simulink model "CPU 4 bit"  (R2022b)
settings: Solver=FixedStepDiscrete  StartTime=0.0  StopTime=10.0  RelTol=1e-3
libraries: hdlsllib x91
settings Model: DataTypeOverride=Off  Creator=canti  LastModifiedBy=canti
settings SolverCC: AlgebraicLoopSolver=TrustRegion
settings DataIOCC: LimitDataPoints=on  SaveOutput=off  SaveTime=off
settings OptimizationCC: BlockReduction=off  ConditionallyExecuteInputs=off  DefaultParameterBehavior=Inlined  LifeSpan=inf
settings DebuggingCC: AlgebraicLoopMsg=error  SingleTaskRateTransMsg=error  UnconnectedInputMsg=warning  UnconnectedOutputMsg=warning  UnconnectedLineMsg=warning  AllowSymbolicDim=off  StrictBusMsg=ErrorOnBusTreatedAsVector  SFUnexpectedBacktrackingDiag=warning  SFNoUnconditionalDefaultTransitionDiag=warning  SFExecutionAtInitializationDiag=none  SFMachineParentedDataDiag=warning  ArithmeticOperatorsInVariantConditions=warning
settings HardwareCC: ProdBitPerPointer=32  ProdBitPerSizeT=32  ProdBitPerPtrDiffT=32  ProdLargestAtomicFloat=None  ProdIntDivRoundTo=Undefined  ProdEndianess=Unspecified  ProdWordSize=32  ProdHWDeviceType=ASIC/FPGA->ASIC/FPGA  ProdEqTarget=off
settings ModelReferenceCC: EnableRefExpFcnMdlSchedulingChecks=on
settings SFSimCC: SimUseLocalCustomCode=off  CustomCodeUndefinedFunction=UseInterfaceOnly
settings RTWCC: RTWUseLocalCustomCode=off
settings CodeAppCC: StateflowObjectComments=on
settings GRTTargetCC: TargetLangStandard=C89/C90 (ANSI)
settings ConfigComp: CovScope=ReferencedModels  CovMetricSettings=dw  CovSaveCumulativeToWorkspaceVar=on  CovSaveSingleToWorkspaceVar=on  CovExternalEMLEnable=off  CovSFcnEnable=off

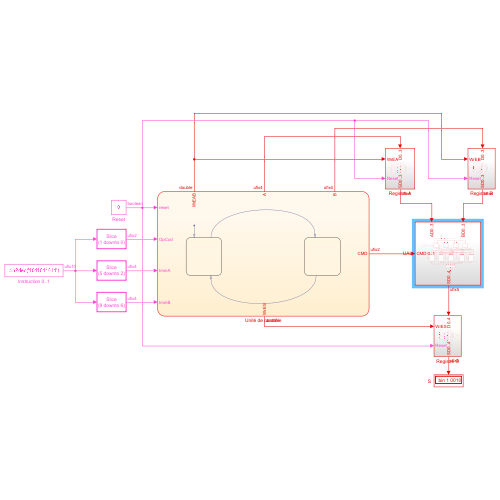
[thumbnail: Simulink's stored preview of the top-level diagram]
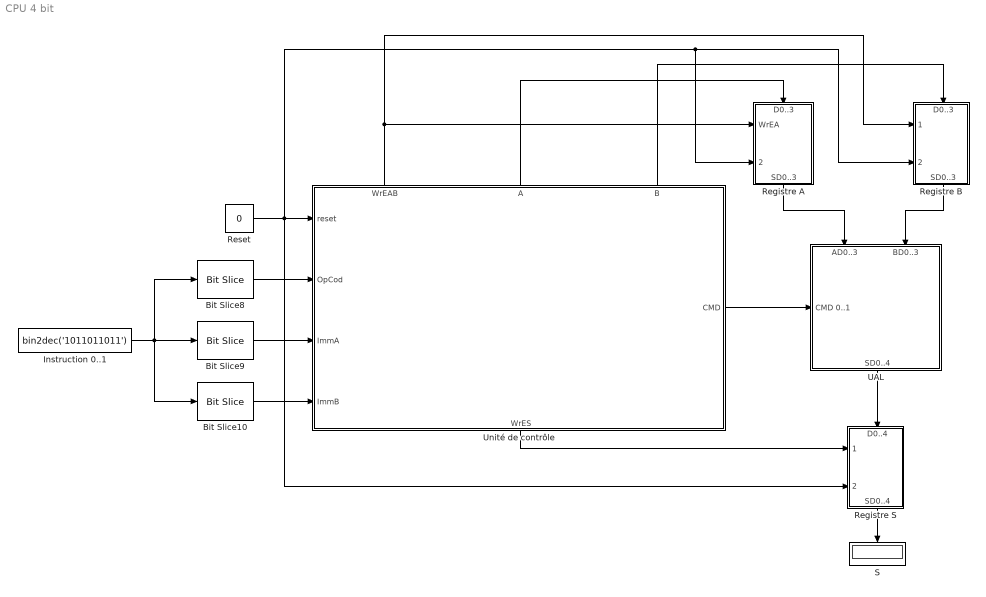
== system CPU 4 bit ==
  Bit Slice10 : hdlsllib/Logic and Bit Operations/Bit Slice  lidx=9  ridx=6
  Bit Slice8 : hdlsllib/Logic and Bit Operations/Bit Slice  lidx=1  ridx=0
  Bit Slice9 : hdlsllib/Logic and Bit Operations/Bit Slice  lidx=5  ridx=2
  Instruction 0..1 : Constant  Value=bin2dec('1011011011')  VectorParams1D=off  OutDataTypeStr=fixdt(0,10,0)
  Registre A : Subsystem
      settings: PortSchema="{\"entries\":[{\"content\":{\"sides\":[{\"content\":{\"connectorIds\":[\"In1\",\"In2\"]},\"type\":\"ConnectorPlacement.EquallySpacedRectSide\",\"uuid\":\"f2a33b33-e521-4072-a478-3afb17db7548\"},{\"content\":{\"connectorIds\":[],\"side\":\"RIGHT\"},\"type\":\"ConnectorPlacement.EquallySpacedRectSide\",\"uuid\":\"da25a38a-bb52-4ad0-9071-b0f3e9d7831e\"},{\"content\":{\"connectorIds\":[\"In3\"],\"side\":\"TOP\"},\"type\":\"ConnectorPlacement.EquallySpacedRectSide\",\"uuid\":\"666d8df1-fd55-45c5-bc82-f8ae5b413d91\"},{\"content\":{\"connectorIds\":[\"Out1\"],\"side\":\"BOTTOM\"},\"type\":\"ConnectorPlacement.EquallySpacedRectSide\",\"uuid\":\"1812bc98-5828-407e-9d5f-9c9edf353f72\"}]},\"type\":\"ConnectorPlacement.EquallySpacedConnector\",\"uuid\":\"1fc978e8-e1f7-4afc-9210-c37bb5433208\"}],\"packageUris\":[\"http://schema.mathworks.com/mf0/Connector/R2020b\"],\"version\":\"1.0\"}"
  Registre B : Subsystem
      settings: PortSchema="{\"entries\":[{\"content\":{\"sides\":[{\"content\":{\"connectorIds\":[\"In1\",\"In2\"]},\"type\":\"ConnectorPlacement.EquallySpacedRectSide\",\"uuid\":\"f2a33b33-e521-4072-a478-3afb17db7548\"},{\"content\":{\"connectorIds\":[],\"side\":\"RIGHT\"},\"type\":\"ConnectorPlacement.EquallySpacedRectSide\",\"uuid\":\"da25a38a-bb52-4ad0-9071-b0f3e9d7831e\"},{\"content\":{\"connectorIds\":[\"In3\"],\"side\":\"TOP\"},\"type\":\"ConnectorPlacement.EquallySpacedRectSide\",\"uuid\":\"666d8df1-fd55-45c5-bc82-f8ae5b413d91\"},{\"content\":{\"connectorIds\":[\"Out1\"],\"side\":\"BOTTOM\"},\"type\":\"ConnectorPlacement.EquallySpacedRectSide\",\"uuid\":\"9285b3be-12c1-44ce-9059-4c76a04c01d8\"}]},\"type\":\"ConnectorPlacement.EquallySpacedConnector\",\"uuid\":\"1fc978e8-e1f7-4afc-9210-c37bb5433208\"}],\"packageUris\":[\"http://schema.mathworks.com/mf0/Connector/R2020b\"],\"version\":\"1.0\"}"
  Registre S : Subsystem
      settings: PortSchema="{\"entries\":[{\"content\":{\"sides\":[{\"content\":{\"connectorIds\":[\"In1\",\"In2\"]},\"type\":\"ConnectorPlacement.EquallySpacedRectSide\",\"uuid\":\"f2a33b33-e521-4072-a478-3afb17db7548\"},{\"content\":{\"connectorIds\":[],\"side\":\"RIGHT\"},\"type\":\"ConnectorPlacement.EquallySpacedRectSide\",\"uuid\":\"da25a38a-bb52-4ad0-9071-b0f3e9d7831e\"},{\"content\":{\"connectorIds\":[\"In3\"],\"side\":\"TOP\"},\"type\":\"ConnectorPlacement.EquallySpacedRectSide\",\"uuid\":\"666d8df1-fd55-45c5-bc82-f8ae5b413d91\"},{\"content\":{\"connectorIds\":[\"Out1\"],\"side\":\"BOTTOM\"},\"type\":\"ConnectorPlacement.EquallySpacedRectSide\",\"uuid\":\"8c02be40-cd01-4bc2-b2ec-2890f76dc57f\"}]},\"type\":\"ConnectorPlacement.EquallySpacedConnector\",\"uuid\":\"1fc978e8-e1f7-4afc-9210-c37bb5433208\"}],\"packageUris\":[\"http://schema.mathworks.com/mf0/Connector/R2020b\"],\"version\":\"1.0\"}"
  Reset : Constant  Value=0  OutDataTypeStr=boolean
  S : Display
      settings: Format=binary (Stored Integer)
  UAL : Subsystem
      settings: PortSchema="{\"entries\":[{\"content\":{\"sides\":[{\"content\":{\"connectorIds\":[\"In1\",\"In2\"]},\"type\":\"ConnectorPlacement.EquallySpacedRectSide\",\"uuid\":\"f2a33b33-e521-4072-a478-3afb17db7548\"},{\"content\":{\"connectorIds\":[\"Out1\"],\"side\":\"RIGHT\"},\"type\":\"ConnectorPlacement.EquallySpacedRectSide\",\"uuid\":\"da25a38a-bb52-4ad0-9071-b0f3e9d7831e\"},{\"content\":{\"connectorIds\":[\"In3\"],\"side\":\"TOP\"},\"type\":\"ConnectorPlacement.EquallySpacedRectSide\",\"uuid\":\"666d8df1-fd55-45c5-bc82-f8ae5b413d91\"}]},\"type\":\"ConnectorPlacement.EquallySpacedConnector\",\"uuid\":\"1fc978e8-e1f7-4afc-9210-c37bb5433208\"}],\"packageUris\":[\"http://schema.mathworks.com/mf0/Connector/R2020b\"],\"version\":\"1.0\"}"
  Unité de contrôle : Stateflow chart  TreatAsAtomicUnit=on
      settings: PortSchema="{\"entries\":[{\"content\":{\"sides\":[{\"content\":{\"connectorIds\":[\"In4\",\"In1\",\"In2\",\"In3\"]},\"type\":\"ConnectorPlacement.EquallySpacedRectSide\",\"uuid\":\"b1c6b50a-e04a-4749-afb5-c5355f577949\"},{\"content\":{\"connectorIds\":[\"Out3\"],\"side\":\"RIGHT\"},\"type\":\"ConnectorPlacement.EquallySpacedRectSide\",\"uuid\":\"2849cef1-e9a5-4d17-bf0d-90818567c808\"},{\"content\":{\"connectorIds\":[\"Out5\",\"Out1\",\"Out2\"],\"side\":\"TOP\"},\"type\":\"ConnectorPlacement.EquallySpacedRectSide\",\"uuid\":\"6f92fd37-1ff9-4600-9dc6-6eccd26e12a7\"},{\"content\":{\"connectorIds\":[\"Out4\"],\"side\":\"BOTTOM\"},\"type\":\"ConnectorPlacement.EquallySpacedRectSide\",\"uuid\":\"4778a550-e515-4b60-9414-e0c210e90663\"}]},\"type\":\"ConnectorPlacement.EquallySpacedConnector\",\"uuid\":\"0744a227-6854-4e56-8184-e9ed60268380\"}],\"packageUris\":[\"http://schema.mathworks.com/mf0/Connector/R2020b\"],\"version\":\"1.0\"}"
  wires:
  Instruction 0..1/1 -> Bit Slice8/1, Bit Slice10/1, Bit Slice9/1
  Reset/1 -> Registre S/2(Reset), Registre B/2(Reset), Registre A/2(Reset), Unité de contrôle/4(reset)
  Bit Slice8/1 -> Unité de contrôle/1(OpCod)
  Bit Slice9/1 -> Unité de contrôle/2(ImmA)
  Bit Slice10/1 -> Unité de contrôle/3(ImmB)
  Unité de contrôle/3(CMD) -> UAL/3(CMD 0..1)
  Unité de contrôle/2(B) -> Registre B/3(D0..3)
  Unité de contrôle/1(A) -> Registre A/3(D0..3)
  Unité de contrôle/5(WrEAB) -> Registre B/1(WrEB), Registre A/1(WrEA)
  Registre A/1(SD0..3) -> UAL/1(AD0..3)
  Registre B/1(SD0..3) -> UAL/2(BD0..3)
  Registre S/1(SD0..4) -> S/1
  Unité de contrôle/4(WrES) -> Registre S/1(WrES)
  UAL/1(SD0..4) -> Registre S/3(D0..4)

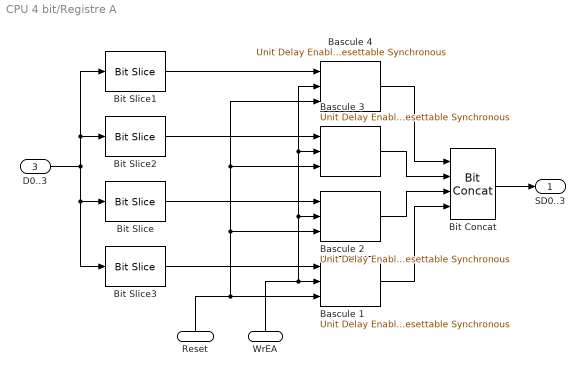
== system CPU 4 bit/Registre A ==
  WrEA : Inport
  Reset : Inport  Port=2
  D0..3 : Inport  Port=3
  Bascule {1..4} (4 alike) : hdlsllib/Discrete/Unit Delay Enabled Resettable Synchronous  InitialCondition=0.0  SampleTime=-1
  Bit Concat : hdlsllib/Logic and Bit Operations/Bit Concat  numInputs=4
  Bit Slice : hdlsllib/Logic and Bit Operations/Bit Slice  lidx=1  ridx=1
  Bit Slice1 : hdlsllib/Logic and Bit Operations/Bit Slice  lidx=3  ridx=3
  Bit Slice2 : hdlsllib/Logic and Bit Operations/Bit Slice  lidx=2  ridx=2
  Bit Slice3 : hdlsllib/Logic and Bit Operations/Bit Slice  lidx=0  ridx=0
  SD0..3 : Outport
  wires:
  WrEA/1 -> Bascule 3/2, Bascule 4/2, Bascule 2/2, Bascule 1/2
  Bit Slice3/1 -> Bascule 1/1
  Reset/1 -> Bascule 4/3, Bascule 3/3, Bascule 2/3, Bascule 1/3
  D0..3/1 -> Bit Slice1/1, Bit Slice2/1, Bit Slice/1, Bit Slice3/1
  Bascule 1/1 -> Bit Concat/4
  Bascule 4/1 -> Bit Concat/1
  Bit Slice2/1 -> Bascule 3/1
  Bit Slice/1 -> Bascule 2/1
  Bit Slice1/1 -> Bascule 4/1
  Bascule 2/1 -> Bit Concat/3
  Bascule 3/1 -> Bit Concat/2
  Bit Concat/1 -> SD0..3/1

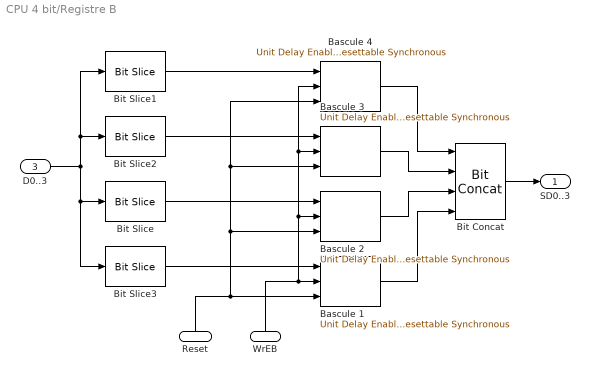
== system CPU 4 bit/Registre B ==
  WrEB : Inport
  Reset : Inport  Port=2
  D0..3 : Inport  Port=3
  Bascule {1..4} (4 alike) : hdlsllib/Discrete/Unit Delay Enabled Resettable Synchronous  InitialCondition=0.0  SampleTime=-1
  Bit Concat : hdlsllib/Logic and Bit Operations/Bit Concat  numInputs=4
  Bit Slice : hdlsllib/Logic and Bit Operations/Bit Slice  lidx=1  ridx=1
  Bit Slice1 : hdlsllib/Logic and Bit Operations/Bit Slice  lidx=3  ridx=3
  Bit Slice2 : hdlsllib/Logic and Bit Operations/Bit Slice  lidx=2  ridx=2
  Bit Slice3 : hdlsllib/Logic and Bit Operations/Bit Slice  lidx=0  ridx=0
  SD0..3 : Outport
  wires:
  WrEB/1 -> Bascule 3/2, Bascule 4/2, Bascule 2/2, Bascule 1/2
  Bit Slice3/1 -> Bascule 1/1
  Reset/1 -> Bascule 4/3, Bascule 3/3, Bascule 2/3, Bascule 1/3
  D0..3/1 -> Bit Slice1/1, Bit Slice2/1, Bit Slice/1, Bit Slice3/1
  Bascule 1/1 -> Bit Concat/4
  Bascule 4/1 -> Bit Concat/1
  Bit Slice2/1 -> Bascule 3/1
  Bit Slice/1 -> Bascule 2/1
  Bit Slice1/1 -> Bascule 4/1
  Bascule 2/1 -> Bit Concat/3
  Bascule 3/1 -> Bit Concat/2
  Bit Concat/1 -> SD0..3/1

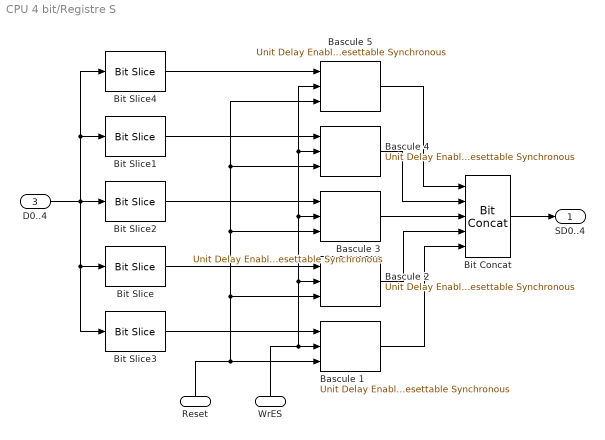
== system CPU 4 bit/Registre S ==
  WrES : Inport
  Reset : Inport  Port=2
  D0..4 : Inport  Port=3
  Bascule {1..5} (5 alike) : hdlsllib/Discrete/Unit Delay Enabled Resettable Synchronous  InitialCondition=0.0  SampleTime=-1
  Bit Concat : hdlsllib/Logic and Bit Operations/Bit Concat  numInputs=5
  Bit Slice : hdlsllib/Logic and Bit Operations/Bit Slice  lidx=1  ridx=1
  Bit Slice1 : hdlsllib/Logic and Bit Operations/Bit Slice  lidx=3  ridx=3
  Bit Slice2 : hdlsllib/Logic and Bit Operations/Bit Slice  lidx=2  ridx=2
  Bit Slice3 : hdlsllib/Logic and Bit Operations/Bit Slice  lidx=0  ridx=0
  Bit Slice4 : hdlsllib/Logic and Bit Operations/Bit Slice  lidx=4  ridx=4
  SD0..4 : Outport
  wires:
  WrES/1 -> Bascule 1/2, Bascule 3/2, Bascule 5/2, Bascule 4/2, Bascule 2/2
  Bit Slice3/1 -> Bascule 1/1
  Reset/1 -> Bascule 5/3, Bascule 4/3, Bascule 3/3, Bascule 2/3, Bascule 1/3
  D0..4/1 -> Bit Slice/1, Bit Slice3/1, Bit Slice4/1, Bit Slice1/1, Bit Slice2/1
  Bit Slice2/1 -> Bascule 3/1
  Bit Slice/1 -> Bascule 2/1
  Bit Slice1/1 -> Bascule 4/1
  Bit Concat/1 -> SD0..4/1
  Bit Slice4/1 -> Bascule 5/1
  Bascule 5/1 -> Bit Concat/1
  Bascule 4/1 -> Bit Concat/2
  Bascule 3/1 -> Bit Concat/3
  Bascule 2/1 -> Bit Concat/4
  Bascule 1/1 -> Bit Concat/5

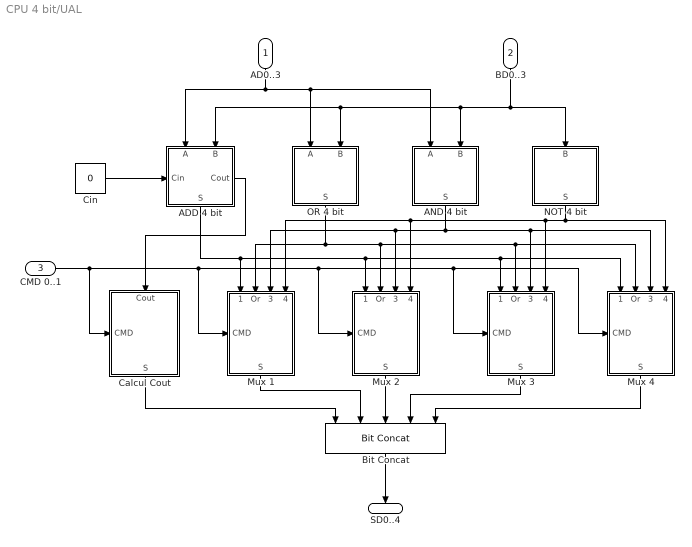
== system CPU 4 bit/UAL ==
  AD0..3 : Inport
  BD0..3 : Inport  Port=2
  CMD 0..1 : Inport  Port=3
  ADD 4 bit : Subsystem
      settings: PortSchema="{\"entries\":[{\"content\":{\"sides\":[{\"content\":{\"connectorIds\":[\"In1\",\"In2\"]},\"type\":\"ConnectorPlacement.EquallySpacedRectSide\",\"uuid\":\"9fdb0751-539c-402b-b5ff-731337fa207a\"},{\"content\":{\"connectorIds\":[\"Out1\"],\"side\":\"RIGHT\"},\"type\":\"ConnectorPlacement.EquallySpacedRectSide\",\"uuid\":\"954d509f-b412-42c8-bfe3-66e195bb53c0\"},{\"content\":{\"connectorIds\":[\"In3\"],\"side\":\"TOP\"},\"type\":\"ConnectorPlacement.EquallySpacedRectSide\",\"uuid\":\"4bbc9f2c-e692-407d-9a36-eff24d7fa996\"},{\"content\":{\"connectorIds\":[\"Out2\"],\"side\":\"BOTTOM\"},\"type\":\"ConnectorPlacement.EquallySpacedRectSide\",\"uuid\":\"365f0ea1-218f-40c9-b891-52372c34a2c2\"}]},\"type\":\"ConnectorPlacement.EquallySpacedConnector\",\"uuid\":\"e3d2d4d1-e117-40a0-87cf-fc38ec024c74\"}],\"packageUris\":[\"http://schema.mathworks.com/mf0/Connector/R2020b\"],\"version\":\"1.0\"}"
  AND 4 bit : Subsystem
  Bit Concat : hdlsllib/Logic and Bit Operations/Bit Concat  numInputs=5
  Calcul Cout : Subsystem
      settings: PortSchema="{\"entries\":[{\"content\":{\"sides\":[{\"content\":{\"connectorIds\":[]},\"type\":\"ConnectorPlacement.EquallySpacedRectSide\",\"uuid\":\"03a4541e-affe-492e-8a0f-e15104ec3d05\"},{\"content\":{\"connectorIds\":[\"In2\"],\"side\":\"RIGHT\"},\"type\":\"ConnectorPlacement.EquallySpacedRectSide\",\"uuid\":\"47fe43af-036d-4db9-a70a-5b35a5803f52\"},{\"content\":{\"connectorIds\":[\"In1\"],\"side\":\"TOP\"},\"type\":\"ConnectorPlacement.EquallySpacedRectSide\",\"uuid\":\"f2e75857-1aa7-44ca-9959-17c78874ce7e\"},{\"content\":{\"connectorIds\":[\"Out1\"],\"side\":\"BOTTOM\"},\"type\":\"ConnectorPlacement.EquallySpacedRectSide\",\"uuid\":\"bd24f4f7-cf2d-42e7-a5b7-ada5d76c273e\"}]},\"type\":\"ConnectorPlacement.EquallySpacedConnector\",\"uuid\":\"5d2b60f3-9ccd-4448-a53a-aff7fd285e89\"}],\"packageUris\":[\"http://schema.mathworks.com/mf0/Connector/R2020b\"],\"version\":\"1.0\"}"
  Cin : Constant  Value=0
  Mux 1 : Subsystem
      settings: PortSchema="{\"entries\":[{\"content\":{\"sides\":[{\"content\":{\"connectorIds\":[\"In1\",\"In2\",\"In3\",\"In4\"]},\"type\":\"ConnectorPlacement.EquallySpacedRectSide\",\"uuid\":\"53602610-42fb-429b-8dfe-dc967cf2471d\"},{\"content\":{\"connectorIds\":[\"Out1\"],\"side\":\"RIGHT\"},\"type\":\"ConnectorPlacement.EquallySpacedRectSide\",\"uuid\":\"8deb7c1e-2f02-4201-bb7e-9ed40c736639\"},{\"content\":{\"connectorIds\":[\"In5\"],\"side\":\"TOP\"},\"type\":\"ConnectorPlacement.EquallySpacedRectSide\",\"uuid\":\"aa45df5f-f144-4bd4-a728-80891a6fc706\"},{\"content\":{\"connectorIds\":[],\"side\":\"BOTTOM\"},\"type\":\"ConnectorPlacement.EquallySpacedRectSide\",\"uuid\":\"ece8f999-6d7b-445a-bb33-5debff738011\"}]},\"type\":\"ConnectorPlacement.EquallySpacedConnector\",\"uuid\":\"c0012ff0-41a7-4b98-bac4-ed1d65952cf4\"}],\"packageUris\":[\"http://schema.mathworks.com/mf0/Connector/R2020b\"],\"version\":\"1.0\"}"
  Mux 2 : Subsystem
      settings: PortSchema="{\"entries\":[{\"content\":{\"sides\":[{\"content\":{\"connectorIds\":[\"In1\",\"In2\",\"In3\",\"In4\"]},\"type\":\"ConnectorPlacement.EquallySpacedRectSide\",\"uuid\":\"53602610-42fb-429b-8dfe-dc967cf2471d\"},{\"content\":{\"connectorIds\":[\"Out1\"],\"side\":\"RIGHT\"},\"type\":\"ConnectorPlacement.EquallySpacedRectSide\",\"uuid\":\"8deb7c1e-2f02-4201-bb7e-9ed40c736639\"},{\"content\":{\"connectorIds\":[\"In5\"],\"side\":\"TOP\"},\"type\":\"ConnectorPlacement.EquallySpacedRectSide\",\"uuid\":\"aa45df5f-f144-4bd4-a728-80891a6fc706\"},{\"content\":{\"connectorIds\":[],\"side\":\"BOTTOM\"},\"type\":\"ConnectorPlacement.EquallySpacedRectSide\",\"uuid\":\"ece8f999-6d7b-445a-bb33-5debff738011\"}]},\"type\":\"ConnectorPlacement.EquallySpacedConnector\",\"uuid\":\"c0012ff0-41a7-4b98-bac4-ed1d65952cf4\"}],\"packageUris\":[\"http://schema.mathworks.com/mf0/Connector/R2020b\"],\"version\":\"1.0\"}"
  Mux 3 : Subsystem
      settings: PortSchema="{\"entries\":[{\"content\":{\"sides\":[{\"content\":{\"connectorIds\":[\"In1\",\"In2\",\"In3\",\"In4\"]},\"type\":\"ConnectorPlacement.EquallySpacedRectSide\",\"uuid\":\"53602610-42fb-429b-8dfe-dc967cf2471d\"},{\"content\":{\"connectorIds\":[\"Out1\"],\"side\":\"RIGHT\"},\"type\":\"ConnectorPlacement.EquallySpacedRectSide\",\"uuid\":\"8deb7c1e-2f02-4201-bb7e-9ed40c736639\"},{\"content\":{\"connectorIds\":[\"In5\"],\"side\":\"TOP\"},\"type\":\"ConnectorPlacement.EquallySpacedRectSide\",\"uuid\":\"aa45df5f-f144-4bd4-a728-80891a6fc706\"},{\"content\":{\"connectorIds\":[],\"side\":\"BOTTOM\"},\"type\":\"ConnectorPlacement.EquallySpacedRectSide\",\"uuid\":\"ece8f999-6d7b-445a-bb33-5debff738011\"}]},\"type\":\"ConnectorPlacement.EquallySpacedConnector\",\"uuid\":\"c0012ff0-41a7-4b98-bac4-ed1d65952cf4\"}],\"packageUris\":[\"http://schema.mathworks.com/mf0/Connector/R2020b\"],\"version\":\"1.0\"}"
  Mux 4 : Subsystem
      settings: PortSchema="{\"entries\":[{\"content\":{\"sides\":[{\"content\":{\"connectorIds\":[\"In1\",\"In2\",\"In3\",\"In4\"]},\"type\":\"ConnectorPlacement.EquallySpacedRectSide\",\"uuid\":\"53602610-42fb-429b-8dfe-dc967cf2471d\"},{\"content\":{\"connectorIds\":[\"Out1\"],\"side\":\"RIGHT\"},\"type\":\"ConnectorPlacement.EquallySpacedRectSide\",\"uuid\":\"8deb7c1e-2f02-4201-bb7e-9ed40c736639\"},{\"content\":{\"connectorIds\":[\"In5\"],\"side\":\"TOP\"},\"type\":\"ConnectorPlacement.EquallySpacedRectSide\",\"uuid\":\"aa45df5f-f144-4bd4-a728-80891a6fc706\"},{\"content\":{\"connectorIds\":[],\"side\":\"BOTTOM\"},\"type\":\"ConnectorPlacement.EquallySpacedRectSide\",\"uuid\":\"ece8f999-6d7b-445a-bb33-5debff738011\"}]},\"type\":\"ConnectorPlacement.EquallySpacedConnector\",\"uuid\":\"c0012ff0-41a7-4b98-bac4-ed1d65952cf4\"}],\"packageUris\":[\"http://schema.mathworks.com/mf0/Connector/R2020b\"],\"version\":\"1.0\"}"
  NOT 4 bit : Subsystem
  OR 4 bit : Subsystem
  SD0..4 : Outport
  wires:
  AD0..3/1 -> AND 4 bit/1(A), OR 4 bit/1(A), ADD 4 bit/1(A)
  BD0..3/1 -> NOT 4 bit/1(B), ADD 4 bit/2(B), OR 4 bit/2(B), AND 4 bit/2(B)
  Bit Concat/1 -> SD0..4/1
  CMD 0..1/1 -> Mux 2/5(CMD), Mux 3/5(CMD), Mux 4/5(CMD), Mux 1/5(CMD), Calcul Cout/2(CMD)
  ADD 4 bit/1(S) -> Mux 2/1(Add), Mux 3/1(Add), Mux 4/1(Add), Mux 1/1(Add)
  OR 4 bit/1(S) -> Mux 3/2(Or), Mux 4/2(Or), Mux 2/2(Or), Mux 1/2(Or)
  AND 4 bit/1(S) -> Mux 3/3(And), Mux 4/3(And), Mux 1/3(And), Mux 2/3(And)
  NOT 4 bit/1(S) -> Mux 4/4(Not), Mux 3/4(Not), Mux 2/4(Not), Mux 1/4(Not)
  Cin/1 -> ADD 4 bit/3(Cin)
  Mux 1/1(S) -> Bit Concat/2
  Mux 2/1(S) -> Bit Concat/3
  Mux 3/1(S) -> Bit Concat/4
  Mux 4/1(S) -> Bit Concat/5
  Calcul Cout/1(S) -> Bit Concat/1
  ADD 4 bit/2(Cout) -> Calcul Cout/1(Cout)

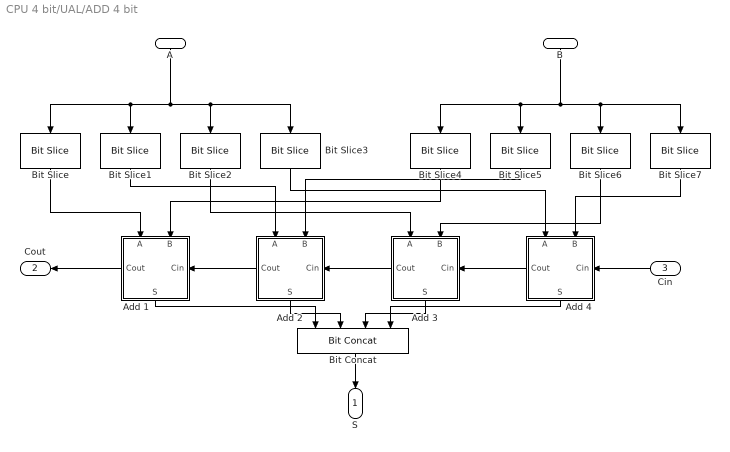
== system CPU 4 bit/UAL/ADD 4 bit ==
  A : Inport
  B : Inport  Port=2
  Cin : Inport  Port=3
  "Add 1 " : Subsystem
      settings: PortSchema="{\"entries\":[{\"content\":{\"sides\":[{\"content\":{\"connectorIds\":[\"In1\",\"In2\"]},\"type\":\"ConnectorPlacement.EquallySpacedRectSide\",\"uuid\":\"19d050e2-e532-41a4-ad1e-957f732a09ea\"},{\"content\":{\"connectorIds\":[\"Out1\"],\"side\":\"RIGHT\"},\"type\":\"ConnectorPlacement.EquallySpacedRectSide\",\"uuid\":\"7f73681e-8ce0-477f-affa-a7014c0263e5\"},{\"content\":{\"connectorIds\":[\"Out2\"],\"side\":\"TOP\"},\"type\":\"ConnectorPlacement.EquallySpacedRectSide\",\"uuid\":\"6a4ba03b-67a4-4950-a6f5-aa10de5d68f9\"},{\"content\":{\"connectorIds\":[\"In3\"],\"side\":\"BOTTOM\"},\"type\":\"ConnectorPlacement.EquallySpacedRectSide\",\"uuid\":\"ba7b3361-7532-4e85-b3d7-908a605896b5\"}]},\"type\":\"ConnectorPlacement.EquallySpacedConnector\",\"uuid\":\"824e3ad9-04be-4ad4-8f26-7228979135e9\"}],\"packageUris\":[\"http://schema.mathworks.com/mf0/Connector/R2020b\"],\"version\":\"1.0\"}"
  Add 2 : Subsystem
      settings: PortSchema="{\"entries\":[{\"content\":{\"sides\":[{\"content\":{\"connectorIds\":[\"In1\",\"In2\"]},\"type\":\"ConnectorPlacement.EquallySpacedRectSide\",\"uuid\":\"19d050e2-e532-41a4-ad1e-957f732a09ea\"},{\"content\":{\"connectorIds\":[\"Out1\"],\"side\":\"RIGHT\"},\"type\":\"ConnectorPlacement.EquallySpacedRectSide\",\"uuid\":\"7f73681e-8ce0-477f-affa-a7014c0263e5\"},{\"content\":{\"connectorIds\":[\"Out2\"],\"side\":\"TOP\"},\"type\":\"ConnectorPlacement.EquallySpacedRectSide\",\"uuid\":\"6a4ba03b-67a4-4950-a6f5-aa10de5d68f9\"},{\"content\":{\"connectorIds\":[\"In3\"],\"side\":\"BOTTOM\"},\"type\":\"ConnectorPlacement.EquallySpacedRectSide\",\"uuid\":\"ba7b3361-7532-4e85-b3d7-908a605896b5\"}]},\"type\":\"ConnectorPlacement.EquallySpacedConnector\",\"uuid\":\"824e3ad9-04be-4ad4-8f26-7228979135e9\"}],\"packageUris\":[\"http://schema.mathworks.com/mf0/Connector/R2020b\"],\"version\":\"1.0\"}"
  Add 3 : Subsystem
      settings: PortSchema="{\"entries\":[{\"content\":{\"sides\":[{\"content\":{\"connectorIds\":[\"In1\",\"In2\"]},\"type\":\"ConnectorPlacement.EquallySpacedRectSide\",\"uuid\":\"19d050e2-e532-41a4-ad1e-957f732a09ea\"},{\"content\":{\"connectorIds\":[\"Out1\"],\"side\":\"RIGHT\"},\"type\":\"ConnectorPlacement.EquallySpacedRectSide\",\"uuid\":\"7f73681e-8ce0-477f-affa-a7014c0263e5\"},{\"content\":{\"connectorIds\":[\"Out2\"],\"side\":\"TOP\"},\"type\":\"ConnectorPlacement.EquallySpacedRectSide\",\"uuid\":\"6a4ba03b-67a4-4950-a6f5-aa10de5d68f9\"},{\"content\":{\"connectorIds\":[\"In3\"],\"side\":\"BOTTOM\"},\"type\":\"ConnectorPlacement.EquallySpacedRectSide\",\"uuid\":\"ba7b3361-7532-4e85-b3d7-908a605896b5\"}]},\"type\":\"ConnectorPlacement.EquallySpacedConnector\",\"uuid\":\"824e3ad9-04be-4ad4-8f26-7228979135e9\"}],\"packageUris\":[\"http://schema.mathworks.com/mf0/Connector/R2020b\"],\"version\":\"1.0\"}"
  Add 4 : Subsystem
      settings: PortSchema="{\"entries\":[{\"content\":{\"sides\":[{\"content\":{\"connectorIds\":[\"In1\",\"In2\"]},\"type\":\"ConnectorPlacement.EquallySpacedRectSide\",\"uuid\":\"19d050e2-e532-41a4-ad1e-957f732a09ea\"},{\"content\":{\"connectorIds\":[\"Out1\"],\"side\":\"RIGHT\"},\"type\":\"ConnectorPlacement.EquallySpacedRectSide\",\"uuid\":\"7f73681e-8ce0-477f-affa-a7014c0263e5\"},{\"content\":{\"connectorIds\":[\"Out2\"],\"side\":\"TOP\"},\"type\":\"ConnectorPlacement.EquallySpacedRectSide\",\"uuid\":\"6a4ba03b-67a4-4950-a6f5-aa10de5d68f9\"},{\"content\":{\"connectorIds\":[\"In3\"],\"side\":\"BOTTOM\"},\"type\":\"ConnectorPlacement.EquallySpacedRectSide\",\"uuid\":\"ba7b3361-7532-4e85-b3d7-908a605896b5\"}]},\"type\":\"ConnectorPlacement.EquallySpacedConnector\",\"uuid\":\"824e3ad9-04be-4ad4-8f26-7228979135e9\"}],\"packageUris\":[\"http://schema.mathworks.com/mf0/Connector/R2020b\"],\"version\":\"1.0\"}"
  Bit Concat : hdlsllib/Logic and Bit Operations/Bit Concat  numInputs=4
  Bit Slice : hdlsllib/Logic and Bit Operations/Bit Slice  lidx=3  ridx=3
  Bit Slice1 : hdlsllib/Logic and Bit Operations/Bit Slice  lidx=2  ridx=2
  Bit Slice2 : hdlsllib/Logic and Bit Operations/Bit Slice  lidx=1  ridx=1
  Bit Slice3 : hdlsllib/Logic and Bit Operations/Bit Slice  lidx=0  ridx=0
  Bit Slice4 : hdlsllib/Logic and Bit Operations/Bit Slice  lidx=3  ridx=3
  Bit Slice5 : hdlsllib/Logic and Bit Operations/Bit Slice  lidx=2  ridx=2
  Bit Slice6 : hdlsllib/Logic and Bit Operations/Bit Slice  lidx=1  ridx=1
  Bit Slice7 : hdlsllib/Logic and Bit Operations/Bit Slice  lidx=0  ridx=0
  S : Outport
  Cout : Outport  Port=2
  wires:
  Bit Slice2/1 -> Add 3/1(" A")
  B/1 -> Bit Slice4/1, Bit Slice5/1, Bit Slice7/1, Bit Slice6/1
  Add 4/1(S) -> Bit Concat/4
  "Add 1 "/1(S) -> Bit Concat/1
  Bit Slice6/1 -> Add 3/2(B)
  Add 3/2(Cout) -> Add 2/3(Cin)
  Add 2/1(S) -> Bit Concat/2
  Bit Slice4/1 -> "Add 1 "/2(B)
  A/1 -> Bit Slice3/1, Bit Slice2/1, Bit Slice1/1, Bit Slice/1
  Add 2/2(Cout) -> "Add 1 "/3(Cin)
  Bit Slice3/1 -> Add 4/1(" A")
  Add 3/1(S) -> Bit Concat/3
  Bit Slice7/1 -> Add 4/2(B)
  Add 4/2(Cout) -> Add 3/3(Cin)
  Bit Slice/1 -> "Add 1 "/1(" A")
  Bit Slice5/1 -> Add 2/2(B)
  Bit Slice1/1 -> Add 2/1(" A")
  Bit Concat/1 -> S/1
  Cin/1 -> Add 4/3(Cin)
  "Add 1 "/2(Cout) -> Cout/1

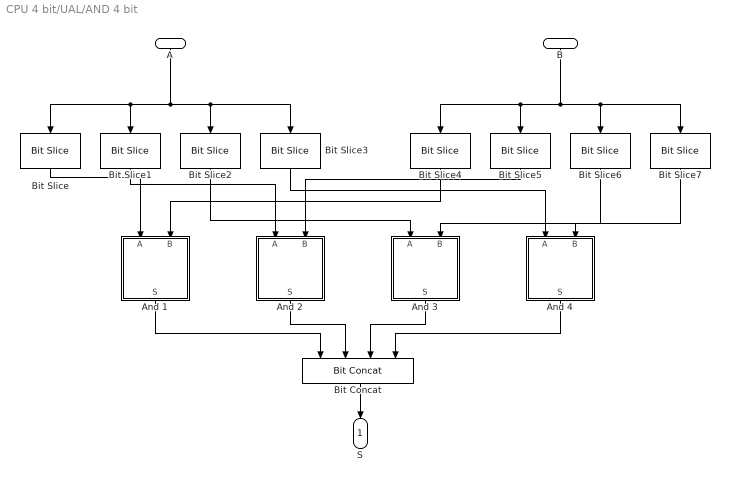
== system CPU 4 bit/UAL/AND 4 bit ==
  A : Inport
  B : Inport  Port=2
  And 1 : Subsystem
  And 2 : Subsystem
  And 3 : Subsystem
  And 4 : Subsystem
  Bit Concat : hdlsllib/Logic and Bit Operations/Bit Concat  numInputs=4
  Bit Slice : hdlsllib/Logic and Bit Operations/Bit Slice  lidx=3  ridx=3
  Bit Slice1 : hdlsllib/Logic and Bit Operations/Bit Slice  lidx=2  ridx=2
  Bit Slice2 : hdlsllib/Logic and Bit Operations/Bit Slice  lidx=1  ridx=1
  Bit Slice3 : hdlsllib/Logic and Bit Operations/Bit Slice  lidx=0  ridx=0
  Bit Slice4 : hdlsllib/Logic and Bit Operations/Bit Slice  lidx=3  ridx=3
  Bit Slice5 : hdlsllib/Logic and Bit Operations/Bit Slice  lidx=2  ridx=2
  Bit Slice6 : hdlsllib/Logic and Bit Operations/Bit Slice  lidx=1  ridx=1
  Bit Slice7 : hdlsllib/Logic and Bit Operations/Bit Slice  lidx=0  ridx=0
  S : Outport
  wires:
  Bit Concat/1 -> S/1
  Bit Slice7/1 -> And 4/2(B)
  Bit Slice3/1 -> And 4/1(" A")
  Bit Slice1/1 -> And 2/1(" A")
  Bit Slice/1 -> And 1/1(" A")
  Bit Slice5/1 -> And 2/2(B)
  A/1 -> Bit Slice3/1, Bit Slice2/1, Bit Slice1/1, Bit Slice/1
  Bit Slice2/1 -> And 3/1(" A")
  And 4/1(S) -> Bit Concat/4
  B/1 -> Bit Slice4/1, Bit Slice5/1, Bit Slice7/1, Bit Slice6/1
  And 1/1(S) -> Bit Concat/1
  Bit Slice4/1 -> And 1/2(B)
  And 2/1(S) -> Bit Concat/2
  And 3/1(S) -> Bit Concat/3
  Bit Slice6/1 -> And 3/2(B)

== system CPU 4 bit/UAL/Calcul Cout ==
  Cout : Inport
  CMD : Inport  Port=2
  Add Cout : Subsystem
  Bit Slice1 : hdlsllib/Logic and Bit Operations/Bit Slice  lidx=1  ridx=1
  Bit Slice2 : hdlsllib/Logic and Bit Operations/Bit Slice  lidx=1  ridx=1
  S : Outport
  wires:
  CMD/1 -> Bit Slice1/1, Bit Slice2/1
  Cout/1 -> Add Cout/3(COUT)
  Bit Slice2/1 -> Add Cout/1(CMD 0)
  Bit Slice1/1 -> Add Cout/2(CMD 1)
  Add Cout/1(S) -> S/1

== system CPU 4 bit/UAL/Mux 1 ==
  Add : Inport
  Or : Inport  Port=2
  And : Inport  Port=3
  Not : Inport  Port=4
  CMD : Inport  Port=5
  Bit Slice{,2..5} (5 alike) : hdlsllib/Logic and Bit Operations/Bit Slice  lidx=0  ridx=0
  Bit Slice1 : hdlsllib/Logic and Bit Operations/Bit Slice  lidx=1  ridx=1
  MUX : Subsystem
      settings: PortSchema="{\"entries\":[{\"content\":{\"sides\":[{\"content\":{\"connectorIds\":[\"In1\",\"In2\",\"In3\",\"In4\"]},\"type\":\"ConnectorPlacement.EquallySpacedRectSide\",\"uuid\":\"528f93b5-72a1-4cc3-864f-1824d66b0a0c\"},{\"content\":{\"connectorIds\":[\"Out1\"],\"side\":\"RIGHT\"},\"type\":\"ConnectorPlacement.EquallySpacedRectSide\",\"uuid\":\"59a09889-0e16-4b9e-86da-a7684ea4f173\"},{\"content\":{\"connectorIds\":[],\"side\":\"TOP\"},\"type\":\"ConnectorPlacement.EquallySpacedRectSide\",\"uuid\":\"e83162ae-8eb8-4b44-ad83-a4c58d87f264\"},{\"content\":{\"connectorIds\":[\"In5\",\"In6\"],\"side\":\"BOTTOM\"},\"type\":\"ConnectorPlacement.EquallySpacedRectSide\",\"uuid\":\"d562e816-dcca-486c-a258-47652e4d677f\"}]},\"type\":\"ConnectorPlacement.EquallySpacedConnector\",\"uuid\":\"101c8411-bd92-428b-95a0-e37421c8efee\"}],\"packageUris\":[\"http://schema.mathworks.com/mf0/Connector/R2020b\"],\"version\":\"1.0\"}"
  S : Outport
  wires:
  And/1 -> Bit Slice4/1
  Add/1 -> Bit Slice2/1
  Or/1 -> Bit Slice3/1
  CMD/1 -> Bit Slice1/1, Bit Slice/1
  Not/1 -> Bit Slice5/1
  Bit Slice2/1 -> MUX/1(Add)
  Bit Slice3/1 -> MUX/2(Or)
  Bit Slice4/1 -> MUX/3(And)
  Bit Slice5/1 -> MUX/4(Not)
  Bit Slice/1 -> MUX/5(CMD 0)
  Bit Slice1/1 -> MUX/6(CMD1)
  MUX/1(S) -> S/1

== system CPU 4 bit/UAL/Mux 2 ==
  Add : Inport
  Or : Inport  Port=2
  And : Inport  Port=3
  Not : Inport  Port=4
  CMD : Inport  Port=5
  Bit Slice : hdlsllib/Logic and Bit Operations/Bit Slice  lidx=0  ridx=0
  Bit Slice{1..5} (5 alike) : hdlsllib/Logic and Bit Operations/Bit Slice  lidx=1  ridx=1
  MUX : Subsystem
      settings: PortSchema="{\"entries\":[{\"content\":{\"sides\":[{\"content\":{\"connectorIds\":[\"In1\",\"In2\",\"In3\",\"In4\"]},\"type\":\"ConnectorPlacement.EquallySpacedRectSide\",\"uuid\":\"528f93b5-72a1-4cc3-864f-1824d66b0a0c\"},{\"content\":{\"connectorIds\":[\"Out1\"],\"side\":\"RIGHT\"},\"type\":\"ConnectorPlacement.EquallySpacedRectSide\",\"uuid\":\"59a09889-0e16-4b9e-86da-a7684ea4f173\"},{\"content\":{\"connectorIds\":[],\"side\":\"TOP\"},\"type\":\"ConnectorPlacement.EquallySpacedRectSide\",\"uuid\":\"e83162ae-8eb8-4b44-ad83-a4c58d87f264\"},{\"content\":{\"connectorIds\":[\"In5\",\"In6\"],\"side\":\"BOTTOM\"},\"type\":\"ConnectorPlacement.EquallySpacedRectSide\",\"uuid\":\"d562e816-dcca-486c-a258-47652e4d677f\"}]},\"type\":\"ConnectorPlacement.EquallySpacedConnector\",\"uuid\":\"101c8411-bd92-428b-95a0-e37421c8efee\"}],\"packageUris\":[\"http://schema.mathworks.com/mf0/Connector/R2020b\"],\"version\":\"1.0\"}"
  S : Outport
  wires:
  And/1 -> Bit Slice4/1
  Add/1 -> Bit Slice2/1
  Or/1 -> Bit Slice3/1
  CMD/1 -> Bit Slice1/1, Bit Slice/1
  Not/1 -> Bit Slice5/1
  Bit Slice2/1 -> MUX/1(Add)
  Bit Slice3/1 -> MUX/2(Or)
  Bit Slice4/1 -> MUX/3(And)
  Bit Slice5/1 -> MUX/4(Not)
  Bit Slice/1 -> MUX/5(CMD 0)
  Bit Slice1/1 -> MUX/6(CMD1)
  MUX/1(S) -> S/1

== system CPU 4 bit/UAL/Mux 3 ==
  Add : Inport
  Or : Inport  Port=2
  And : Inport  Port=3
  Not : Inport  Port=4
  CMD : Inport  Port=5
  Bit Slice : hdlsllib/Logic and Bit Operations/Bit Slice  lidx=0  ridx=0
  Bit Slice1 : hdlsllib/Logic and Bit Operations/Bit Slice  lidx=1  ridx=1
  Bit Slice{2..5} (4 alike) : hdlsllib/Logic and Bit Operations/Bit Slice  lidx=2  ridx=2
  MUX : Subsystem
      settings: PortSchema="{\"entries\":[{\"content\":{\"sides\":[{\"content\":{\"connectorIds\":[\"In1\",\"In2\",\"In3\",\"In4\"]},\"type\":\"ConnectorPlacement.EquallySpacedRectSide\",\"uuid\":\"528f93b5-72a1-4cc3-864f-1824d66b0a0c\"},{\"content\":{\"connectorIds\":[\"Out1\"],\"side\":\"RIGHT\"},\"type\":\"ConnectorPlacement.EquallySpacedRectSide\",\"uuid\":\"59a09889-0e16-4b9e-86da-a7684ea4f173\"},{\"content\":{\"connectorIds\":[],\"side\":\"TOP\"},\"type\":\"ConnectorPlacement.EquallySpacedRectSide\",\"uuid\":\"e83162ae-8eb8-4b44-ad83-a4c58d87f264\"},{\"content\":{\"connectorIds\":[\"In5\",\"In6\"],\"side\":\"BOTTOM\"},\"type\":\"ConnectorPlacement.EquallySpacedRectSide\",\"uuid\":\"d562e816-dcca-486c-a258-47652e4d677f\"}]},\"type\":\"ConnectorPlacement.EquallySpacedConnector\",\"uuid\":\"101c8411-bd92-428b-95a0-e37421c8efee\"}],\"packageUris\":[\"http://schema.mathworks.com/mf0/Connector/R2020b\"],\"version\":\"1.0\"}"
  S : Outport
  wires:
  And/1 -> Bit Slice4/1
  Add/1 -> Bit Slice2/1
  Or/1 -> Bit Slice3/1
  CMD/1 -> Bit Slice1/1, Bit Slice/1
  Not/1 -> Bit Slice5/1
  Bit Slice2/1 -> MUX/1(Add)
  Bit Slice3/1 -> MUX/2(Or)
  Bit Slice4/1 -> MUX/3(And)
  Bit Slice5/1 -> MUX/4(Not)
  Bit Slice/1 -> MUX/5(CMD 0)
  Bit Slice1/1 -> MUX/6(CMD1)
  MUX/1(S) -> S/1

== system CPU 4 bit/UAL/Mux 4 ==
  Add : Inport
  Or : Inport  Port=2
  And : Inport  Port=3
  Not : Inport  Port=4
  CMD : Inport  Port=5
  Bit Slice : hdlsllib/Logic and Bit Operations/Bit Slice  lidx=0  ridx=0
  Bit Slice1 : hdlsllib/Logic and Bit Operations/Bit Slice  lidx=1  ridx=1
  Bit Slice{2..5} (4 alike) : hdlsllib/Logic and Bit Operations/Bit Slice  lidx=3  ridx=3
  MUX : Subsystem
      settings: PortSchema="{\"entries\":[{\"content\":{\"sides\":[{\"content\":{\"connectorIds\":[\"In1\",\"In2\",\"In3\",\"In4\"]},\"type\":\"ConnectorPlacement.EquallySpacedRectSide\",\"uuid\":\"528f93b5-72a1-4cc3-864f-1824d66b0a0c\"},{\"content\":{\"connectorIds\":[\"Out1\"],\"side\":\"RIGHT\"},\"type\":\"ConnectorPlacement.EquallySpacedRectSide\",\"uuid\":\"59a09889-0e16-4b9e-86da-a7684ea4f173\"},{\"content\":{\"connectorIds\":[],\"side\":\"TOP\"},\"type\":\"ConnectorPlacement.EquallySpacedRectSide\",\"uuid\":\"e83162ae-8eb8-4b44-ad83-a4c58d87f264\"},{\"content\":{\"connectorIds\":[\"In5\",\"In6\"],\"side\":\"BOTTOM\"},\"type\":\"ConnectorPlacement.EquallySpacedRectSide\",\"uuid\":\"d562e816-dcca-486c-a258-47652e4d677f\"}]},\"type\":\"ConnectorPlacement.EquallySpacedConnector\",\"uuid\":\"101c8411-bd92-428b-95a0-e37421c8efee\"}],\"packageUris\":[\"http://schema.mathworks.com/mf0/Connector/R2020b\"],\"version\":\"1.0\"}"
  S : Outport
  wires:
  And/1 -> Bit Slice4/1
  Add/1 -> Bit Slice2/1
  Or/1 -> Bit Slice3/1
  CMD/1 -> Bit Slice1/1, Bit Slice/1
  Not/1 -> Bit Slice5/1
  Bit Slice2/1 -> MUX/1(Add)
  Bit Slice3/1 -> MUX/2(Or)
  Bit Slice4/1 -> MUX/3(And)
  Bit Slice5/1 -> MUX/4(Not)
  Bit Slice/1 -> MUX/5(CMD 0)
  Bit Slice1/1 -> MUX/6(CMD1)
  MUX/1(S) -> S/1

== system CPU 4 bit/UAL/NOT 4 bit ==
  B : Inport
  Bit Concat : hdlsllib/Logic and Bit Operations/Bit Concat  numInputs=4
  Bit Slice4 : hdlsllib/Logic and Bit Operations/Bit Slice  lidx=3  ridx=3
  Bit Slice5 : hdlsllib/Logic and Bit Operations/Bit Slice  lidx=2  ridx=2
  Bit Slice6 : hdlsllib/Logic and Bit Operations/Bit Slice  lidx=1  ridx=1
  Bit Slice7 : hdlsllib/Logic and Bit Operations/Bit Slice  lidx=0  ridx=0
  Not 1 : Subsystem
  Not 2 : Subsystem
  Not 3 : Subsystem
  Not 4 : Subsystem
  S : Outport
  wires:
  Bit Concat/1 -> S/1
  Bit Slice7/1 -> Not 4/1(B)
  Bit Slice5/1 -> Not 2/1(B)
  Not 4/1(S) -> Bit Concat/4
  B/1 -> Bit Slice4/1, Bit Slice5/1, Bit Slice7/1, Bit Slice6/1
  Not 1/1(S) -> Bit Concat/1
  Bit Slice4/1 -> Not 1/1(B)
  Not 2/1(S) -> Bit Concat/2
  Not 3/1(S) -> Bit Concat/3
  Bit Slice6/1 -> Not 3/1(B)

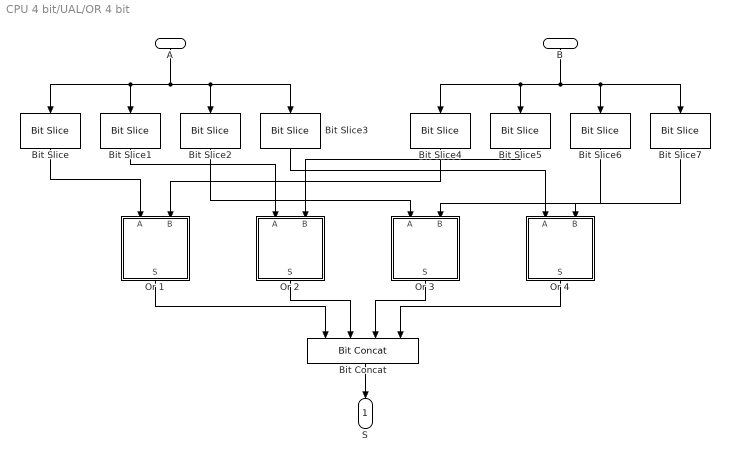
== system CPU 4 bit/UAL/OR 4 bit ==
  A : Inport
  B : Inport  Port=2
  Bit Concat : hdlsllib/Logic and Bit Operations/Bit Concat  numInputs=4
  Bit Slice : hdlsllib/Logic and Bit Operations/Bit Slice  lidx=3  ridx=3
  Bit Slice1 : hdlsllib/Logic and Bit Operations/Bit Slice  lidx=2  ridx=2
  Bit Slice2 : hdlsllib/Logic and Bit Operations/Bit Slice  lidx=1  ridx=1
  Bit Slice3 : hdlsllib/Logic and Bit Operations/Bit Slice  lidx=0  ridx=0
  Bit Slice4 : hdlsllib/Logic and Bit Operations/Bit Slice  lidx=3  ridx=3
  Bit Slice5 : hdlsllib/Logic and Bit Operations/Bit Slice  lidx=2  ridx=2
  Bit Slice6 : hdlsllib/Logic and Bit Operations/Bit Slice  lidx=1  ridx=1
  Bit Slice7 : hdlsllib/Logic and Bit Operations/Bit Slice  lidx=0  ridx=0
  Or 1 : Subsystem
  Or 2 : Subsystem
  Or 3 : Subsystem
  Or 4 : Subsystem
  S : Outport
  wires:
  Bit Concat/1 -> S/1
  Bit Slice7/1 -> Or 4/2(B)
  Bit Slice3/1 -> Or 4/1(" A")
  Bit Slice1/1 -> Or 2/1(" A")
  Bit Slice/1 -> Or 1/1(" A")
  Bit Slice5/1 -> Or 2/2(B)
  A/1 -> Bit Slice3/1, Bit Slice2/1, Bit Slice1/1, Bit Slice/1
  Bit Slice2/1 -> Or 3/1(" A")
  Or 4/1(S) -> Bit Concat/4
  B/1 -> Bit Slice4/1, Bit Slice5/1, Bit Slice7/1, Bit Slice6/1
  Or 1/1(S) -> Bit Concat/1
  Bit Slice4/1 -> Or 1/2(B)
  Or 2/1(S) -> Bit Concat/2
  Or 3/1(S) -> Bit Concat/3
  Bit Slice6/1 -> Or 3/2(B)

== system CPU 4 bit/UAL/ADD 4 bit/Add 1  ==
  " A" : Inport
  B : Inport  Port=2
  Cin : Inport  Port=3
  AND : Logic  IconShape=distinctive  AllPortsSameDT=off  OutDataTypeStr=boolean
  AND1 : Logic  IconShape=distinctive  AllPortsSameDT=off  OutDataTypeStr=boolean
  XOR : Logic  Operator=XOR  IconShape=distinctive  AllPortsSameDT=off  OutDataTypeStr=boolean
  XOR1 : Logic  Operator=XOR  IconShape=distinctive  AllPortsSameDT=off  OutDataTypeStr=boolean
  XOR2 : Logic  Operator=XOR  IconShape=distinctive  AllPortsSameDT=off  OutDataTypeStr=boolean
  S : Outport
  Cout : Outport  Port=2
  wires:
  " A"/1 -> XOR/1, AND1/2
  XOR/1 -> AND/2, XOR1/1
  B/1 -> AND1/1, XOR/2
  Cin/1 -> AND/1, XOR1/2
  AND/1 -> XOR2/1
  XOR2/1 -> Cout/1
  AND1/1 -> XOR2/2
  XOR1/1 -> S/1

== system CPU 4 bit/UAL/ADD 4 bit/Add 2 ==
  " A" : Inport
  B : Inport  Port=2
  Cin : Inport  Port=3
  AND : Logic  IconShape=distinctive  AllPortsSameDT=off  OutDataTypeStr=boolean
  AND1 : Logic  IconShape=distinctive  AllPortsSameDT=off  OutDataTypeStr=boolean
  XOR : Logic  Operator=XOR  IconShape=distinctive  AllPortsSameDT=off  OutDataTypeStr=boolean
  XOR1 : Logic  Operator=XOR  IconShape=distinctive  AllPortsSameDT=off  OutDataTypeStr=boolean
  XOR2 : Logic  Operator=XOR  IconShape=distinctive  AllPortsSameDT=off  OutDataTypeStr=boolean
  S : Outport
  Cout : Outport  Port=2
  wires:
  " A"/1 -> XOR/1, AND1/2
  XOR/1 -> AND/2, XOR1/1
  B/1 -> AND1/1, XOR/2
  Cin/1 -> AND/1, XOR1/2
  AND/1 -> XOR2/1
  XOR2/1 -> Cout/1
  AND1/1 -> XOR2/2
  XOR1/1 -> S/1

== system CPU 4 bit/UAL/ADD 4 bit/Add 3 ==
  " A" : Inport
  B : Inport  Port=2
  Cin : Inport  Port=3
  AND : Logic  IconShape=distinctive  AllPortsSameDT=off  OutDataTypeStr=boolean
  AND1 : Logic  IconShape=distinctive  AllPortsSameDT=off  OutDataTypeStr=boolean
  XOR : Logic  Operator=XOR  IconShape=distinctive  AllPortsSameDT=off  OutDataTypeStr=boolean
  XOR1 : Logic  Operator=XOR  IconShape=distinctive  AllPortsSameDT=off  OutDataTypeStr=boolean
  XOR2 : Logic  Operator=XOR  IconShape=distinctive  AllPortsSameDT=off  OutDataTypeStr=boolean
  S : Outport
  Cout : Outport  Port=2
  wires:
  " A"/1 -> XOR/1, AND1/2
  XOR/1 -> AND/2, XOR1/1
  B/1 -> AND1/1, XOR/2
  Cin/1 -> AND/1, XOR1/2
  AND/1 -> XOR2/1
  XOR2/1 -> Cout/1
  AND1/1 -> XOR2/2
  XOR1/1 -> S/1

== system CPU 4 bit/UAL/ADD 4 bit/Add 4 ==
  " A" : Inport
  B : Inport  Port=2
  Cin : Inport  Port=3
  AND : Logic  IconShape=distinctive  AllPortsSameDT=off  OutDataTypeStr=boolean
  AND1 : Logic  IconShape=distinctive  AllPortsSameDT=off  OutDataTypeStr=boolean
  XOR : Logic  Operator=XOR  IconShape=distinctive  AllPortsSameDT=off  OutDataTypeStr=boolean
  XOR1 : Logic  Operator=XOR  IconShape=distinctive  AllPortsSameDT=off  OutDataTypeStr=boolean
  XOR2 : Logic  Operator=XOR  IconShape=distinctive  AllPortsSameDT=off  OutDataTypeStr=boolean
  S : Outport
  Cout : Outport  Port=2
  wires:
  " A"/1 -> XOR/1, AND1/2
  XOR/1 -> AND/2, XOR1/1
  B/1 -> AND1/1, XOR/2
  Cin/1 -> AND/1, XOR1/2
  AND/1 -> XOR2/1
  XOR2/1 -> Cout/1
  AND1/1 -> XOR2/2
  XOR1/1 -> S/1

== system CPU 4 bit/UAL/AND 4 bit/And 1 ==
  " A" : Inport
  B : Inport  Port=2
  XOR : Logic  IconShape=distinctive  AllPortsSameDT=off  OutDataTypeStr=boolean
  S : Outport
  wires:
  " A"/1 -> XOR/1
  B/1 -> XOR/2
  XOR/1 -> S/1

== system CPU 4 bit/UAL/AND 4 bit/And 2 ==
  " A" : Inport
  B : Inport  Port=2
  XOR : Logic  IconShape=distinctive  AllPortsSameDT=off  OutDataTypeStr=boolean
  S : Outport
  wires:
  " A"/1 -> XOR/1
  B/1 -> XOR/2
  XOR/1 -> S/1

== system CPU 4 bit/UAL/AND 4 bit/And 3 ==
  " A" : Inport
  B : Inport  Port=2
  XOR : Logic  IconShape=distinctive  AllPortsSameDT=off  OutDataTypeStr=boolean
  S : Outport
  wires:
  " A"/1 -> XOR/1
  B/1 -> XOR/2
  XOR/1 -> S/1

== system CPU 4 bit/UAL/AND 4 bit/And 4 ==
  " A" : Inport
  B : Inport  Port=2
  XOR : Logic  IconShape=distinctive  AllPortsSameDT=off  OutDataTypeStr=boolean
  S : Outport
  wires:
  " A"/1 -> XOR/1
  B/1 -> XOR/2
  XOR/1 -> S/1

== system CPU 4 bit/UAL/Calcul Cout/Add Cout ==
  CMD 0 : Inport
  CMD 1 : Inport  Port=2
  COUT : Inport  Port=3
  AND : Logic  Inputs=3  IconShape=distinctive  AllPortsSameDT=off  OutDataTypeStr=boolean
  S : Outport
  wires:
  AND/1 -> S/1
  CMD 1/1 -> AND/2
  CMD 0/1 -> AND/1
  COUT/1 -> AND/3

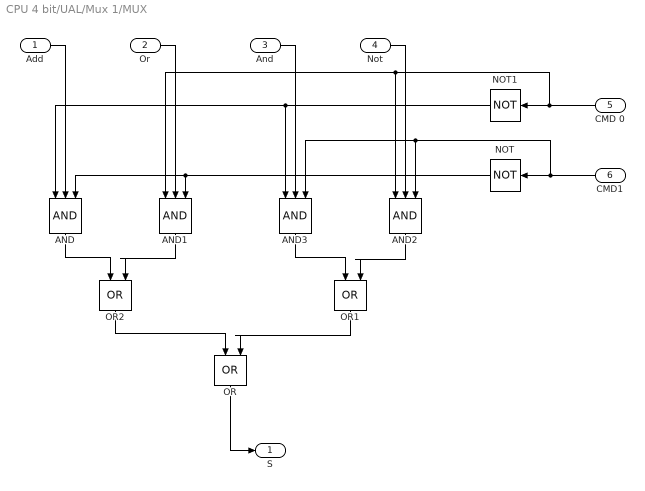
== system CPU 4 bit/UAL/Mux 1/MUX ==
  Add : Inport
  Or : Inport  Port=2
  And : Inport  Port=3
  Not : Inport  Port=4
  CMD 0 : Inport  Port=5
  CMD1 : Inport  Port=6
  AND{,1..3} (4 alike) : Logic  Inputs=3  IconShape=distinctive  AllPortsSameDT=off  OutDataTypeStr=boolean
  NOT : Logic  Operator=NOT  IconShape=distinctive  AllPortsSameDT=off  OutDataTypeStr=boolean
  NOT1 : Logic  Operator=NOT  IconShape=distinctive  AllPortsSameDT=off  OutDataTypeStr=boolean
  OR : Logic  Operator=OR  IconShape=distinctive  AllPortsSameDT=off  OutDataTypeStr=boolean
  OR1 : Logic  Operator=OR  IconShape=distinctive  AllPortsSameDT=off  OutDataTypeStr=boolean
  OR2 : Logic  Operator=OR  IconShape=distinctive  AllPortsSameDT=off  OutDataTypeStr=boolean
  S : Outport
  wires:
  AND/1 -> OR2/1
  NOT/1 -> AND/3, AND1/3
  CMD1/1 -> NOT/1, AND2/3, AND3/3
  CMD 0/1 -> AND1/1, AND2/1, NOT1/1
  NOT1/1 -> AND/1, AND3/1
  Or/1 -> AND1/2
  OR2/1 -> OR/1
  AND1/1 -> OR2/2
  Add/1 -> AND/2
  AND2/1 -> OR1/2
  OR/1 -> S/1
  OR1/1 -> OR/2
  AND3/1 -> OR1/1
  And/1 -> AND3/2
  Not/1 -> AND2/2

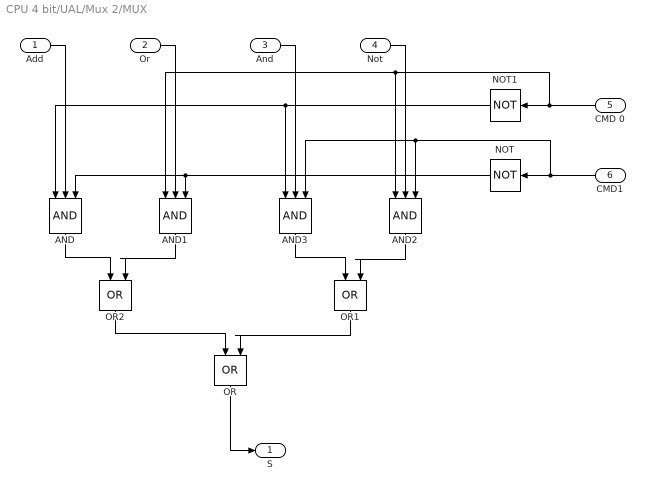
== system CPU 4 bit/UAL/Mux 2/MUX ==
  Add : Inport
  Or : Inport  Port=2
  And : Inport  Port=3
  Not : Inport  Port=4
  CMD 0 : Inport  Port=5
  CMD1 : Inport  Port=6
  AND{,1..3} (4 alike) : Logic  Inputs=3  IconShape=distinctive  AllPortsSameDT=off  OutDataTypeStr=boolean
  NOT : Logic  Operator=NOT  IconShape=distinctive  AllPortsSameDT=off  OutDataTypeStr=boolean
  NOT1 : Logic  Operator=NOT  IconShape=distinctive  AllPortsSameDT=off  OutDataTypeStr=boolean
  OR : Logic  Operator=OR  IconShape=distinctive  AllPortsSameDT=off  OutDataTypeStr=boolean
  OR1 : Logic  Operator=OR  IconShape=distinctive  AllPortsSameDT=off  OutDataTypeStr=boolean
  OR2 : Logic  Operator=OR  IconShape=distinctive  AllPortsSameDT=off  OutDataTypeStr=boolean
  S : Outport
  wires:
  AND/1 -> OR2/1
  NOT/1 -> AND/3, AND1/3
  CMD1/1 -> NOT/1, AND2/3, AND3/3
  CMD 0/1 -> AND1/1, AND2/1, NOT1/1
  NOT1/1 -> AND/1, AND3/1
  Or/1 -> AND1/2
  OR2/1 -> OR/1
  AND1/1 -> OR2/2
  Add/1 -> AND/2
  AND2/1 -> OR1/2
  OR/1 -> S/1
  OR1/1 -> OR/2
  AND3/1 -> OR1/1
  And/1 -> AND3/2
  Not/1 -> AND2/2

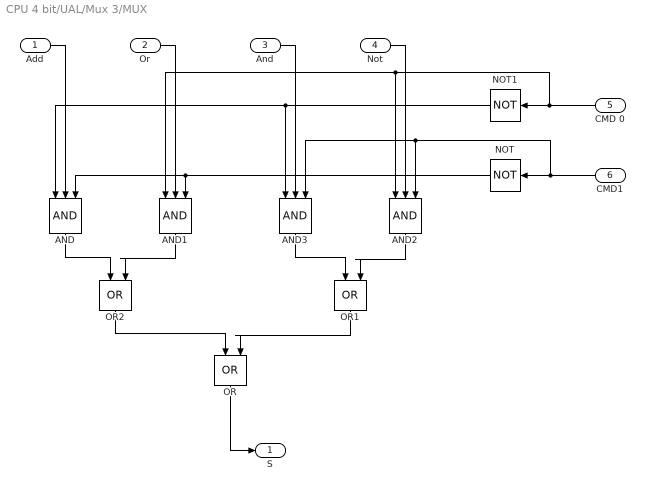
== system CPU 4 bit/UAL/Mux 3/MUX ==
  Add : Inport
  Or : Inport  Port=2
  And : Inport  Port=3
  Not : Inport  Port=4
  CMD 0 : Inport  Port=5
  CMD1 : Inport  Port=6
  AND{,1..3} (4 alike) : Logic  Inputs=3  IconShape=distinctive  AllPortsSameDT=off  OutDataTypeStr=boolean
  NOT : Logic  Operator=NOT  IconShape=distinctive  AllPortsSameDT=off  OutDataTypeStr=boolean
  NOT1 : Logic  Operator=NOT  IconShape=distinctive  AllPortsSameDT=off  OutDataTypeStr=boolean
  OR : Logic  Operator=OR  IconShape=distinctive  AllPortsSameDT=off  OutDataTypeStr=boolean
  OR1 : Logic  Operator=OR  IconShape=distinctive  AllPortsSameDT=off  OutDataTypeStr=boolean
  OR2 : Logic  Operator=OR  IconShape=distinctive  AllPortsSameDT=off  OutDataTypeStr=boolean
  S : Outport
  wires:
  AND/1 -> OR2/1
  NOT/1 -> AND/3, AND1/3
  CMD1/1 -> NOT/1, AND2/3, AND3/3
  CMD 0/1 -> AND1/1, AND2/1, NOT1/1
  NOT1/1 -> AND/1, AND3/1
  Or/1 -> AND1/2
  OR2/1 -> OR/1
  AND1/1 -> OR2/2
  Add/1 -> AND/2
  AND2/1 -> OR1/2
  OR/1 -> S/1
  OR1/1 -> OR/2
  AND3/1 -> OR1/1
  And/1 -> AND3/2
  Not/1 -> AND2/2

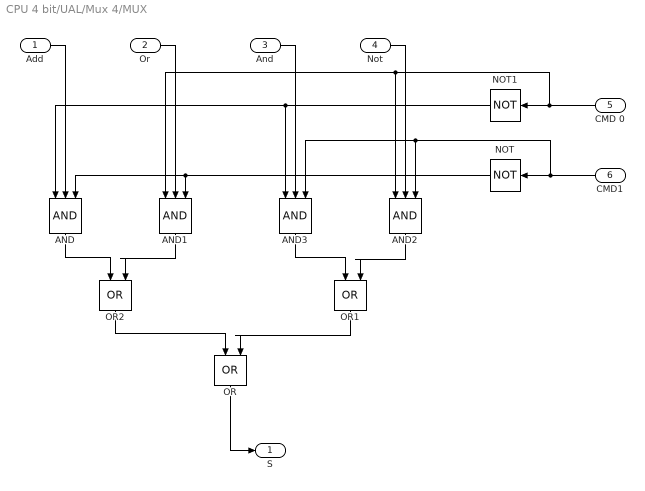
== system CPU 4 bit/UAL/Mux 4/MUX ==
  Add : Inport
  Or : Inport  Port=2
  And : Inport  Port=3
  Not : Inport  Port=4
  CMD 0 : Inport  Port=5
  CMD1 : Inport  Port=6
  AND{,1..3} (4 alike) : Logic  Inputs=3  IconShape=distinctive  AllPortsSameDT=off  OutDataTypeStr=boolean
  NOT : Logic  Operator=NOT  IconShape=distinctive  AllPortsSameDT=off  OutDataTypeStr=boolean
  NOT1 : Logic  Operator=NOT  IconShape=distinctive  AllPortsSameDT=off  OutDataTypeStr=boolean
  OR : Logic  Operator=OR  IconShape=distinctive  AllPortsSameDT=off  OutDataTypeStr=boolean
  OR1 : Logic  Operator=OR  IconShape=distinctive  AllPortsSameDT=off  OutDataTypeStr=boolean
  OR2 : Logic  Operator=OR  IconShape=distinctive  AllPortsSameDT=off  OutDataTypeStr=boolean
  S : Outport
  wires:
  AND/1 -> OR2/1
  NOT/1 -> AND/3, AND1/3
  CMD1/1 -> NOT/1, AND2/3, AND3/3
  CMD 0/1 -> AND1/1, AND2/1, NOT1/1
  NOT1/1 -> AND/1, AND3/1
  Or/1 -> AND1/2
  OR2/1 -> OR/1
  AND1/1 -> OR2/2
  Add/1 -> AND/2
  AND2/1 -> OR1/2
  OR/1 -> S/1
  OR1/1 -> OR/2
  AND3/1 -> OR1/1
  And/1 -> AND3/2
  Not/1 -> AND2/2

== system CPU 4 bit/UAL/NOT 4 bit/Not 1 ==
  B : Inport
  NOT : Logic  Operator=NOT  IconShape=distinctive  AllPortsSameDT=off  OutDataTypeStr=boolean
  S : Outport
  wires:
  B/1 -> NOT/1
  NOT/1 -> S/1

== system CPU 4 bit/UAL/NOT 4 bit/Not 2 ==
  B : Inport
  NOT : Logic  Operator=NOT  IconShape=distinctive  AllPortsSameDT=off  OutDataTypeStr=boolean
  S : Outport
  wires:
  B/1 -> NOT/1
  NOT/1 -> S/1

== system CPU 4 bit/UAL/NOT 4 bit/Not 3 ==
  B : Inport
  NOT : Logic  Operator=NOT  IconShape=distinctive  AllPortsSameDT=off  OutDataTypeStr=boolean
  S : Outport
  wires:
  B/1 -> NOT/1
  NOT/1 -> S/1

== system CPU 4 bit/UAL/NOT 4 bit/Not 4 ==
  B : Inport
  NOT : Logic  Operator=NOT  IconShape=distinctive  AllPortsSameDT=off  OutDataTypeStr=boolean
  S : Outport
  wires:
  B/1 -> NOT/1
  NOT/1 -> S/1

== system CPU 4 bit/UAL/OR 4 bit/Or 1 ==
  " A" : Inport
  B : Inport  Port=2
  XOR : Logic  Operator=OR  IconShape=distinctive  AllPortsSameDT=off  OutDataTypeStr=boolean
  S : Outport
  wires:
  " A"/1 -> XOR/1
  B/1 -> XOR/2
  XOR/1 -> S/1

== system CPU 4 bit/UAL/OR 4 bit/Or 2 ==
  " A" : Inport
  B : Inport  Port=2
  XOR : Logic  Operator=OR  IconShape=distinctive  AllPortsSameDT=off  OutDataTypeStr=boolean
  S : Outport
  wires:
  " A"/1 -> XOR/1
  B/1 -> XOR/2
  XOR/1 -> S/1

== system CPU 4 bit/UAL/OR 4 bit/Or 3 ==
  " A" : Inport
  B : Inport  Port=2
  XOR : Logic  Operator=OR  IconShape=distinctive  AllPortsSameDT=off  OutDataTypeStr=boolean
  S : Outport
  wires:
  " A"/1 -> XOR/1
  B/1 -> XOR/2
  XOR/1 -> S/1

== system CPU 4 bit/UAL/OR 4 bit/Or 4 ==
  " A" : Inport
  B : Inport  Port=2
  XOR : Logic  Operator=OR  IconShape=distinctive  AllPortsSameDT=off  OutDataTypeStr=boolean
  S : Outport
  wires:
  " A"/1 -> XOR/1
  B/1 -> XOR/2
  XOR/1 -> S/1

== stateflow chart CPU 4 bit/Unité de contrôle ==
  state Initial
    A=ImmA
    B=ImmB
    CMD=OpCod
  state Cours
    A=ImmA
    B=ImmB
    CMD=OpCod
    WrES=1
    WrEAB=1
  Initial -> Cours : [reset == 0]
  (default) -> Initial
  Cours -> Initial : [reset == 1]
  data: OpCod input; ImmA input; A output; B output; CMD output; WrES output; WrEAB output; ImmB input; reset input
